simulink model "offGrid_Inverter"  (R2022b)
settings: Solver=FixedStepDiscrete  StartTime=0.0  StopTime=2  FixedStep=1e-6  RelTol=1e-3
libraries: spsSeriesRLCBranchLib x11, spsCurrentMeasurementLib x7, spsMosfetLib x6, slpidlib x5, spsRMSLib x4, simulink x4, spsFourierLib x2, spsTriangleGeneratorLib x2, spsVoltageMeasurementLib x2, spsBreakerLib x1, spsDCVoltageSourceLib x1, spspowerguiLib x1
(part 2 of 2)

== matlab function offGrid_Inverter/MATLAB Function5 ==
  data: I_ref input; duty_out output; I_fb input
function duty_out = fcn(I_ref, I_fb)
%#codegen
% 同步Boost电流环PI控制器（带钳位抗饱和）
% 适配：20kHz采样、±5A电流传感器、占空比0.1~0.9安全范围
% 输入：
%   I_ref: 电压环输出的电流给定（对应你模型里电压环PI的输出）
%   I_fb: 电流反馈（对应你模型里经过-1增益后的IL信号）
% 输出：
%   duty_out: 最终占空比，直接接你模型里的1/z延迟模块

% 持久化变量：保存积分器状态，每个控制周期保留数值
persistent integral_val;
% 初始化：仅仿真启动的第一个控制周期执行1次
if isempty(integral_val)
    integral_val = 0;
end

% ==================== 1. 控制参数（和你原PI模块参数完全一致，可直接修改）====================
Kp = 0.05;       % 比例增益，和你原设置一致
Ki = 10;         % 积分增益，和你原设置一致
Ts = 5e-5;       % 20kHz控制周期，固定不变
% ==================== 2. 物理极限设置（核心抗饱和阈值）====================
DUTY_MAX = 0.57;  % 占空比上限，避免上下管直通
DUTY_MIN = 0.15;  % 占空比下限，杜绝轻载反向电流
I_SAT_LIMIT = 5.0; % 电流传感器饱和阈值，接近±5A量程提前触发保护

% ==================== 3. 误差计算 ====================
err = I_ref - I_fb;

% ==================== 4. 比例项输出 ====================
prop_out = Kp * err;

% ==================== 5. 核心抗饱和逻辑 ====================
% 5.1 积分项预计算
integral_inc = Ki * Ts * err;
integral_pre = integral_val + integral_inc;
% 5.2 预计算不饱和的PI输出
duty_pre = prop_out + integral_pre;

% 5.3 钳位抗饱和规则：
% 仅当输出在线性区、且电流未达到传感器饱和阈值时，才允许积分累加
% 同时加入反向积分放行规则，避免积分锁死
is_duty_linear = (duty_pre < DUTY_MAX) && (duty_pre > DUTY_MIN);
is_current_unsat = (abs(I_fb) < I_SAT_LIMIT);
is_integral_allow = is_duty_linear && is_current_unsat;
is_reverse_integral = (err > 0 && integral_pre < 0) || (err < 0 && integral_pre > 0);

if is_integral_allow || is_reverse_integral
    integral_val = integral_pre;
end

% ==================== 6. 最终占空比计算 + 硬限幅兜底 ====================
duty_out = prop_out + integral_val;
duty_out = min(max(duty_out, DUTY_MIN), DUTY_MAX);

== matlab function offGrid_Inverter/MATLAB Function6 ==
  data: t input; y output
function y = smooth_rise(t)
% 功能：输入时间t，输出1秒内从0线性增长到32
% 线性上升（无曲线，匀速增长）

T = 1;    % 上升时间 1 秒
A = 32;   % 目标值

if t < 0
    y = 0;
elseif t <= T
    % 线性上升公式
    y = A * (t / T);  
else
    y = A;
end
end

== matlab function offGrid_Inverter/MATLAB Function7 ==
  data: t input; v_ref output
function v_ref = fcn(t)
    % 定义参数
    V_start = 34.0;  % 起始电压
    V_end = 55.0;    % 目标电压
    T_ramp = 1.0;    % 增长持续时间 (秒)
    
    % 逻辑判断
    if t <= 0
        % 仿真开始前或瞬时，保持起始值
        v_ref = V_start;
    elseif t >= T_ramp
        % 1秒之后，保持在55V
        v_ref = V_end;
    else
        % 0s 到 1s 之间线性增长
        % 公式：起始值 + (电压差 / 时间差) * 当前时间
        v_ref = V_start + (V_end - V_start) * (t / T_ramp);
    end
end

== matlab function offGrid_Inverter/重复控制1 ==
  data: u_in input; u_out output
function u_out = Repetitive_Controller_Internal_Param(u_in)
%REPETITIVE_CONTROLLER_Internal_Param 内部可修改参数的重复控制器
% 功能：
%   可直接在函数内部修改 p、k_rc、N 三个核心参数
%   修复「变量b未完全定义」错误，适配Simulink Coder
% 采样周期：Ts = 1e-4 s（10kHz）

%% ===================== 预定义全局变量（解决未定义错误） =====================
% 提前初始化所有变量，覆盖所有执行路径
persistent x b a;   % 状态变量+系数变量
if isempty(x)
    %% ===================== 1. 在这里修改你的参数 =====================
    N = 400;          % 基波周期采样次数（可改）   采样频率/基波频率
    p = 3;            % 相位补偿阶数（可改，例如 p=5）
    k_rc = 0.3;       % 收敛系数（可改，例如 0.3/0.5）
    % ================================================================

    %% ===================== 2. 固定参数 Q(z) = 0.25z + 0.5 + 0.25/z =====================
    Q0 = 0.25;
    Q1 = 0.5;
    Q2 = 0.25;

    %% ===================== 3. 计算延迟阶数 =====================
    delay_order = N - p;  % 分子延迟阶数 = z^(-delay_order)

    %% ===================== 4. 构造分子和分母（显式离散计算） =====================
    max_order = N + 2;    % 统一最大阶数：N+2

    % 强制初始化分子/分母（覆盖所有执行路径）
    b = zeros(1, max_order + 1);  % z降幂：z^0 ~ z^(-max_order)
    a = zeros(1, max_order + 1);
    a(1) = 1.0;  % 分母首项=1

    % 填入分子系数（强制赋值，无分支）
    b(delay_order + 3) = k_rc * Q2;  % z^(-(delay_order+2))
    b(delay_order + 2) = k_rc * Q1;  % z^(-(delay_order+1))
    b(delay_order + 1) = k_rc * Q0;  % z^(-delay_order)

    % 填入分母系数（强制赋值，无分支）
    a(N + 1) = a(N + 1) - Q0;  % z^(-N)
    a(N + 2) = a(N + 2) - Q1;  % z^(-(N+1))
    a(N + 3) = a(N + 3) - Q2;  % z^(-(N+2))

    %% ===================== 5. 初始化状态变量 =====================
    x = zeros(length(a) - 1, 1);
end

%% ===================== 6. 直接II型差分方程（实时计算） =====================
% 输出计算（确保b的长度匹配x）
u_out = b(1) * u_in;
if length(b) > 1
    for i = 2:length(b)
        if i-1 <= length(x)
            u_out = u_out + b(i) * x(i-1);
        end
    end
end

% 状态更新（逐行实现，避免dot函数）
for n = 1:length(x)-1
    x(n) = b(n+1)*u_in - a(n+1)*u_out + x(n+1);
end
x(end) = b(end)*u_in - a(end)*u_out;

end



% function u_out = Repetitive_Controller_Internal_Param(u_in)
% REPETITIVE_CONTROLLER_Internal_Param Q=0.9常数版重复控制器
% 功能：
%   Q(z)固定为0.9常数（无二阶滤波），仅保留重复控制核心延迟环节
%   可修改 p、k_rc、N 三个核心参数，适配Simulink Coder
% 采样周期：Ts = 1e-4 s（10kHz）
% 
% % ===================== 预定义全局变量（解决未定义错误） =====================
% persistent x b a;   % 状态变量+系数变量
% if isempty(x)
%     % ===================== 1. 核心参数配置（可修改） =====================
%     N = 200;          % 基波周期采样次数（50Hz基波，10kHz采样→N=200）
%     p = 3;            % 相位补偿阶数
%     k_rc = 0.41;      % 收敛系数
%     Q = 0.9;          % 固定低通常数（替代原二阶Q(z)）
%     ================================================================
% 
%     % ===================== 2. 计算延迟阶数 =====================
%     delay_order = N - p;  % 分子延迟阶数 = z^(-delay_order)
% 
%     % ===================== 3. 构造分子和分母（常数Q版） =====================
%     max_order = N;       % 简化最大阶数（仅保留N阶延迟，无额外滤波阶数）
% 
%     强制初始化分子/分母（覆盖所有执行路径）
%     b = zeros(1, max_order + 1);  % z降幂：z^0 ~ z^(-max_order)
%     a = zeros(1, max_order + 1);
%     a(1) = 1.0;  % 分母首项=1
% 
%     填入分子系数（仅保留常数Q的延迟项）
%     b(delay_order + 1) = k_rc * Q;  % 分子：k_rc * Q * z^(-delay_order)
% 
%     填入分母系数（仅保留常数Q的N阶延迟项）
%     a(N + 1) = a(N + 1) - Q;       % 分母：1 - Q * z^(-N)
% 
%     % ===================== 4. 初始化状态变量 =====================
%     x = zeros(length(a) - 1, 1);  % 状态变量长度=分母阶数
% end
% 
% % ===================== 5. 直接II型差分方程（实时计算） =====================
% 输出计算（确保b的长度匹配x）
% u_out = b(1) * u_in;
% if length(b) > 1
%     for i = 2:length(b)
%         if i-1 <= length(x)
%             u_out = u_out + b(i) * x(i-1);
%         end
%     end
% end
% 
% 状态更新（逐行实现，避免dot函数，适配代码生成）
% for n = 1:length(x)-1
%     x(n) = b(n+1)*u_in - a(n+1)*u_out + x(n+1);
% end
% x(end) = b(end)*u_in - a(end)*u_out;
% 
% end
% 
% 
% 
% 
%

== matlab function offGrid_Inverter/MATLAB Function8 ==
  data: I_ref input; duty_out output; I_fb input
function duty_out = fcn(I_ref, I_fb)
%#codegen
% 同步Boost电流环PI控制器（带钳位抗饱和）
% 适配：20kHz采样、±5A电流传感器、占空比0.1~0.9安全范围
% 输入：
%   I_ref: 电压环输出的电流给定（对应你模型里电压环PI的输出）
%   I_fb: 电流反馈（对应你模型里经过-1增益后的IL信号）
% 输出：
%   duty_out: 最终占空比，直接接你模型里的1/z延迟模块

% 持久化变量：保存积分器状态，每个控制周期保留数值
persistent integral_val;
% 初始化：仅仿真启动的第一个控制周期执行1次
if isempty(integral_val)
    integral_val = 0;
end

% ==================== 1. 控制参数（和你原PI模块参数完全一致，可直接修改）====================
Kp = 0.05;       % 比例增益，和你原设置一致
Ki = 8600;         % 积分增益，和你原设置一致
Ts = 5e-5;       % 20kHz控制周期，固定不变
% ==================== 2. 物理极限设置（核心抗饱和阈值）====================
DUTY_MAX = 1000;  % 占空比上限，避免上下管直通
DUTY_MIN = -1000;  % 占空比下限，杜绝轻载反向电流
I_SAT_LIMIT = 50.0; % 电流传感器饱和阈值，接近±5A量程提前触发保护

% ==================== 3. 误差计算 ====================
err = I_ref - I_fb;

% ==================== 4. 比例项输出 ====================
prop_out = Kp * err;

% ==================== 5. 核心抗饱和逻辑 ====================
% 5.1 积分项预计算
integral_inc = Ki * Ts * err;
integral_pre = integral_val + integral_inc;
% 5.2 预计算不饱和的PI输出
duty_pre = prop_out + integral_pre;

% 5.3 钳位抗饱和规则：
% 仅当输出在线性区、且电流未达到传感器饱和阈值时，才允许积分累加
% 同时加入反向积分放行规则，避免积分锁死
is_duty_linear = (duty_pre < DUTY_MAX) && (duty_pre > DUTY_MIN);
is_current_unsat = (abs(I_fb) < I_SAT_LIMIT);
is_integral_allow = is_duty_linear && is_current_unsat;
is_reverse_integral = (err > 0 && integral_pre < 0) || (err < 0 && integral_pre > 0);

if is_integral_allow || is_reverse_integral
    integral_val = integral_pre;
end

% ==================== 6. 最终占空比计算 + 硬限幅兜底 ====================
duty_out = prop_out + integral_val;
duty_out = min(max(duty_out, DUTY_MIN), DUTY_MAX);

== matlab function offGrid_Inverter/MATLAB Function1 ==
  data: t input; y output
function y = smooth_rise(t)
% 功能：输入时间t，输出0.3秒内从0平滑曲线增长到32
% 曲线类型：余弦缓升（无超调、无冲击，工业控制标准）
% 规则：
%   t < 0        → 输出 0
%   0 ≤ t ≤ 0.3s → 平滑从 0 增长到 32
%   t > 0.3s     → 保持 32

T = 0.3;   % 总上升时间 0.3秒
A = 32;    % 目标值

if t < 0
    y = 0;
elseif t <= T
    % 余弦平滑增长公式
    tau = t / T;
    smooth_curve = 0.5 * (1 - cos(pi * tau));
    y = A * smooth_curve;
else
    y = A;
end
end

== matlab function offGrid_Inverter/MATLAB Function9 ==
  data: I_ref input; duty_out output; I_fb input
function duty_out = fcn(I_ref, I_fb)
%#codegen
% 同步Boost电流环PI控制器（带钳位抗饱和）
% 适配：20kHz采样、±5A电流传感器、占空比0.1~0.9安全范围
% 输入：
%   I_ref: 电压环输出的电流给定（对应你模型里电压环PI的输出）
%   I_fb: 电流反馈（对应你模型里经过-1增益后的IL信号）
% 输出：
%   duty_out: 最终占空比，直接接你模型里的1/z延迟模块

% 持久化变量：保存积分器状态，每个控制周期保留数值
persistent integral_val;
% 初始化：仅仿真启动的第一个控制周期执行1次
if isempty(integral_val)
    integral_val = 0;
end

% ==================== 1. 控制参数（和你原PI模块参数完全一致，可直接修改）====================
Kp = 0.1;       % 比例增益，和你原设置一致
Ki = 0;         % 积分增益，和你原设置一致
Ts = 5e-5;       % 20kHz控制周期，固定不变
% ==================== 2. 物理极限设置（核心抗饱和阈值）====================
DUTY_MAX = 0.9;  % 占空比上限，避免上下管直通
DUTY_MIN = -0.9;  % 占空比下限，杜绝轻载反向电流
I_SAT_LIMIT = 10.0; % 电流传感器饱和阈值，接近±5A量程提前触发保护

% ==================== 3. 误差计算 ====================
err = I_ref - I_fb;

% ==================== 4. 比例项输出 ====================
prop_out = Kp * err;

% ==================== 5. 核心抗饱和逻辑 ====================
% 5.1 积分项预计算
integral_inc = Ki * Ts * err;
integral_pre = integral_val + integral_inc;
% 5.2 预计算不饱和的PI输出
duty_pre = prop_out + integral_pre;

% 5.3 钳位抗饱和规则：
% 仅当输出在线性区、且电流未达到传感器饱和阈值时，才允许积分累加
% 同时加入反向积分放行规则，避免积分锁死
is_duty_linear = (duty_pre < DUTY_MAX) && (duty_pre > DUTY_MIN);
is_current_unsat = (abs(I_fb) < I_SAT_LIMIT);
is_integral_allow = is_duty_linear && is_current_unsat;
is_reverse_integral = (err > 0 && integral_pre < 0) || (err < 0 && integral_pre > 0);

if is_integral_allow || is_reverse_integral
    integral_val = integral_pre;
end

% ==================== 6. 最终占空比计算 + 硬限幅兜底 ====================
duty_out = prop_out + integral_val;
duty_out = min(max(duty_out, DUTY_MIN), DUTY_MAX);

== matlab function offGrid_Inverter/正确版本的重复控制（计算量大） ==
  data: u_in input; u_out output
function u_out = Repetitive_Controller_Internal_Param(u_in)
%REPETITIVE_CONTROLLER_Internal_Param 内部可修改参数的重复控制器
% 功能：
%   可直接在函数内部修改 p、k_rc、N 三个核心参数
%   修复「变量b未完全定义」错误，适配Simulink Coder
% 采样周期：Ts = 1e-4 s（10kHz）

%% ===================== 预定义全局变量（解决未定义错误） =====================
% 提前初始化所有变量，覆盖所有执行路径
persistent x b a;   % 状态变量+系数变量
if isempty(x)
    %% ===================== 1. 在这里修改你的参数 =====================
    N = 400;          % 基波周期采样次数（可改）   采样频率/基波频率
    p = 3;            % 相位补偿阶数（可改，例如 p=5）
    k_rc = 0.3;       % 收敛系数（可改，例如 0.3/0.5）
    % ================================================================

    %% ===================== 2. 固定参数 Q(z) = 0.25z + 0.5 + 0.25/z =====================
    Q0 = 0.25;
    Q1 = 0.5;
    Q2 = 0.25;

    %% ===================== 3. 计算延迟阶数 =====================
    delay_order = N - p;  % 分子延迟阶数 = z^(-delay_order)

    %% ===================== 4. 构造分子和分母（显式离散计算） =====================
    max_order = N + 2;    % 统一最大阶数：N+2

    % 强制初始化分子/分母（覆盖所有执行路径）
    b = zeros(1, max_order + 1);  % z降幂：z^0 ~ z^(-max_order)
    a = zeros(1, max_order + 1);
    a(1) = 1.0;  % 分母首项=1

    % 填入分子系数（强制赋值，无分支）
    b(delay_order + 3) = k_rc * Q2;  % z^(-(delay_order+2))
    b(delay_order + 2) = k_rc * Q1;  % z^(-(delay_order+1))
    b(delay_order + 1) = k_rc * Q0;  % z^(-delay_order)

    % 填入分母系数（强制赋值，无分支）
    a(N + 1) = a(N + 1) - Q0;  % z^(-N)
    a(N + 2) = a(N + 2) - Q1;  % z^(-(N+1))
    a(N + 3) = a(N + 3) - Q2;  % z^(-(N+2))

    %% ===================== 5. 初始化状态变量 =====================
    x = zeros(length(a) - 1, 1);
end

%% ===================== 6. 直接II型差分方程（实时计算） =====================
% 输出计算（确保b的长度匹配x）
u_out = b(1) * u_in;
if length(b) > 1
    for i = 2:length(b)
        if i-1 <= length(x)
            u_out = u_out + b(i) * x(i-1);
        end
    end
end

% 状态更新（逐行实现，避免dot函数）
for n = 1:length(x)-1
    x(n) = b(n+1)*u_in - a(n+1)*u_out + x(n+1);
end
x(end) = b(end)*u_in - a(end)*u_out;

end



% function u_out = Repetitive_Controller_Internal_Param(u_in)
% REPETITIVE_CONTROLLER_Internal_Param Q=0.9常数版重复控制器
% 功能：
%   Q(z)固定为0.9常数（无二阶滤波），仅保留重复控制核心延迟环节
%   可修改 p、k_rc、N 三个核心参数，适配Simulink Coder
% 采样周期：Ts = 1e-4 s（10kHz）
% 
% % ===================== 预定义全局变量（解决未定义错误） =====================
% persistent x b a;   % 状态变量+系数变量
% if isempty(x)
%     % ===================== 1. 核心参数配置（可修改） =====================
%     N = 200;          % 基波周期采样次数（50Hz基波，10kHz采样→N=200）
%     p = 3;            % 相位补偿阶数
%     k_rc = 0.41;      % 收敛系数
%     Q = 0.9;          % 固定低通常数（替代原二阶Q(z)）
%     ================================================================
% 
%     % ===================== 2. 计算延迟阶数 =====================
%     delay_order = N - p;  % 分子延迟阶数 = z^(-delay_order)
% 
%     % ===================== 3. 构造分子和分母（常数Q版） =====================
%     max_order = N;       % 简化最大阶数（仅保留N阶延迟，无额外滤波阶数）
% 
%     强制初始化分子/分母（覆盖所有执行路径）
%     b = zeros(1, max_order + 1);  % z降幂：z^0 ~ z^(-max_order)
%     a = zeros(1, max_order + 1);
%     a(1) = 1.0;  % 分母首项=1
% 
%     填入分子系数（仅保留常数Q的延迟项）
%     b(delay_order + 1) = k_rc * Q;  % 分子：k_rc * Q * z^(-delay_order)
% 
%     填入分母系数（仅保留常数Q的N阶延迟项）
%     a(N + 1) = a(N + 1) - Q;       % 分母：1 - Q * z^(-N)
% 
%     % ===================== 4. 初始化状态变量 =====================
%     x = zeros(length(a) - 1, 1);  % 状态变量长度=分母阶数
% end
% 
% % ===================== 5. 直接II型差分方程（实时计算） =====================
% 输出计算（确保b的长度匹配x）
% u_out = b(1) * u_in;
% if length(b) > 1
%     for i = 2:length(b)
%         if i-1 <= length(x)
%             u_out = u_out + b(i) * x(i-1);
%         end
%     end
% end
% 
% 状态更新（逐行实现，避免dot函数，适配代码生成）
% for n = 1:length(x)-1
%     x(n) = b(n+1)*u_in - a(n+1)*u_out + x(n+1);
% end
% x(end) = b(end)*u_in - a(end)*u_out;
% 
% end
% 
% 
% 
% 
%

== matlab function offGrid_Inverter/rc滤波1 ==
  data: u input; y output
function y = fcn(u)
% 一阶RC低通滤波（数字等效实现）
% 适配：仿真步长 Ts=1e-6s（Fs=1MHz），截止频率 fc=4.7kHz
% 输入：u - 原始信号
% 输出：y - RC滤波后的信号

% persistent 变量保存上一时刻的输出（RC滤波的状态）
persistent y_prev;

% ---------------- 固定参数（已按你的需求预计算） ----------------
fc = 4700;   % 截止频率：4.7kHz
Ts = 1e-6;   % 仿真步长：1us（1e-6s）
tau = 1/(2*pi*fc); % RC时间常数 τ=RC=1/(2πfc)
alpha = exp(-Ts/tau); % 滤波系数（RC离散化核心）
% ----------------------------------------------------------------

% 初始化状态（仅第一次调用时执行，默认初始输出为0）
if isempty(y_prev)
    y_prev = 0;
end

% 一阶RC低通的离散差分方程（和真实RC电路特性完全等效）
y = alpha * y_prev + (1 - alpha) * u;

% 更新状态，为下一个仿真步准备
y_prev = y;

end
